simulink model "MPC_Regulator"  (R2022a)
settings: Solver=VariableStepAuto  StartTime=0.0  StopTime=20.0  RelTol=1e-3
settings Model: Creator=caoya  LastModifiedBy=caoya

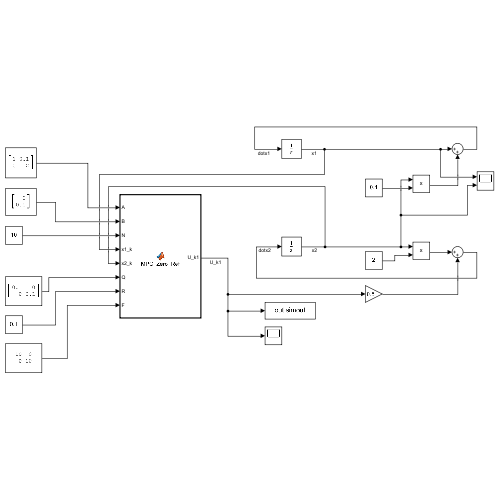
[thumbnail: Simulink's stored preview of the top-level diagram]
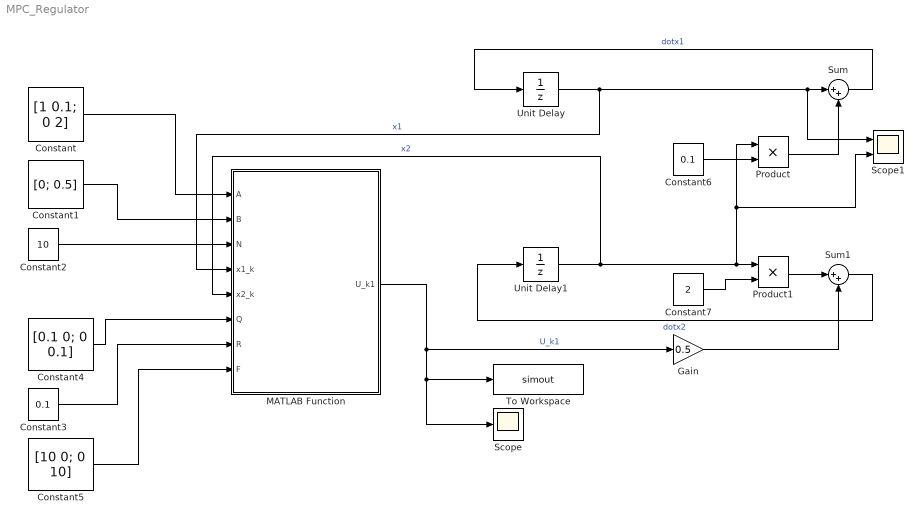
== system MPC_Regulator ==
  Constant : Constant  Value=[1 0.1; 0 2]
  Constant1 : Constant  Value=[0; 0.5]  VectorParams1D=off
  Constant2 : Constant  Value=10
  Constant3 : Constant  Value=0.1
  Constant4 : Constant  Value=[0.1 0; 0 0.1]
  Constant5 : Constant  Value=[10 0; 0 10]
  Constant6 : Constant  Value=0.1
  Constant7 : Constant  Value=2
  Gain : Gain  Gain=0.5
  MATLAB Function : MATLAB Function  TreatAsAtomicUnit=on
  Product : Product
  Product1 : Product
  Scope : Scope
  Scope1 : Scope  NumInputPorts=2
  Sum : Sum  Inputs=|++
  Sum1 : Sum  Inputs=|++
  To Workspace : ToWorkspace  VariableName=simout  SaveFormat=Timeseries  SampleTime=-1
  Unit Delay : UnitDelay  InitialCondition=5  SampleTime=-1  HasFrameUpgradeWarning=on
  Unit Delay1 : UnitDelay  InitialCondition=5  SampleTime=-1  HasFrameUpgradeWarning=on
  wires:
  Constant/1 -> MATLAB Function/1(A)
  Constant1/1 -> MATLAB Function/2(B)
  Constant2/1 -> MATLAB Function/3(N)
  Constant3/1 -> MATLAB Function/7(R)
  Constant4/1 -> MATLAB Function/6(Q)
  Constant5/1 -> MATLAB Function/8(F)
  Constant6/1 -> Product/2
  Unit Delay1/1 -> MATLAB Function/5(x2_k), Product1/1, Scope1/2, Product/1  "x2"
  Product/1 -> Sum/2
  Sum/1 -> Unit Delay/1  "dotx1"
  Constant7/1 -> Product1/2
  Product1/1 -> Sum1/1
  Gain/1 -> Sum1/2
  MATLAB Function/1(U_k1) -> Scope/1, To Workspace/1, Gain/1  "U_k1"
  Sum1/1 -> Unit Delay1/1  "dotx2"
  Unit Delay/1 -> MATLAB Function/4(x1_k), Scope1/1, Sum/1  "x1"

== matlab function MPC_Regulator/MATLAB Function ==
  data: A input; B input; N input; x1_k input; x2_k input; Q input; R input; F input; U_k1 output
function U_k1  = MPC_Zero_Ref(A, B, N, x1_k, x2_k, Q, R, F)
coder.extrinsic('quadprog');
U_k1 = zeros(1, 1);

% find the dimensions of A and B
n = size(A, 1);           % A is a nxn matrix
p = size(B, 2);           % B is a nxp matrix

% initialize C, it is a (N)
% the upper part is a nxn I, the lower part is firstly defined as 0
M = [eye(n); zeros(N * n, n)];

% initialize C, a (N+1)n x Np matrix firstly with 0
C = zeros((N + 1) * n, N * p);

% define M and C
tmp = eye(n);
for i = 1: N
    % define current row, begin with i * n, and have n rows in total
    rows = i * n + (1: n);
    % fill C
    C(rows, :) = [tmp * B, C(rows-n, 1: end-p)];
    % Each time tmp left multiplys A
    tmp = A * tmp;

    % fill M
    M(rows, :) = tmp;
end

% define Q_bar
% find the dimensions of Q and R
S_q = size(Q, 1);
S_r = size(R, 1);
% initialize Q_bar with 0
Q_bar = zeros((N + 1)*S_q, (N+1)*S_q);
% arrange Q onto the diagonal
for i = 0: N-1
    Q_bar(i * S_q + 1: (i + 1) * S_q, i*S_q + 1: (i + 1) * S_q) = Q;
end
% put F in the last place
Q_bar((N - 1) * S_q + 1: N * S_q, (N - 1) * S_q + 1: N * S_q) = F;

% define R_bar
R_bar = zeros(N * S_r, N * S_r);
for i = 0: N - 1
    R_bar(i * S_r + 1: (i + 1) * S_r, i * S_r + 1: (i + 1) * S_r) = R;
end

% solve G, E, H
G = M' * Q_bar * M;
E = M' * Q_bar * C;
H = C' * Q_bar * C + R_bar;

% optimal control
% define x_k
x_k = [x1_k; x2_k];
% define f
f = (x_k' * E)';
% solve the optimal U_k
U_k = quadprog(H, f);
U_k1 = U_k(1);

end
